simulink model "FA_18_Model"  (R2018a)
settings: Solver=ode45  StartTime=0.0  StopTime=20  FixedStep=0.1  MaxStep=0.1  RelTol=1e-3
PreLoadFcn:
  | load('FA_18_Parameters.mat')
  | format long
undefined symbols (not defined in the file or in its folder): Earth, WGS84
libraries: aerolibfltsims x1, aerolibtransform2 x1, aerolibconvert2 x1
settings Model: Creator=User  LastModifiedBy=User

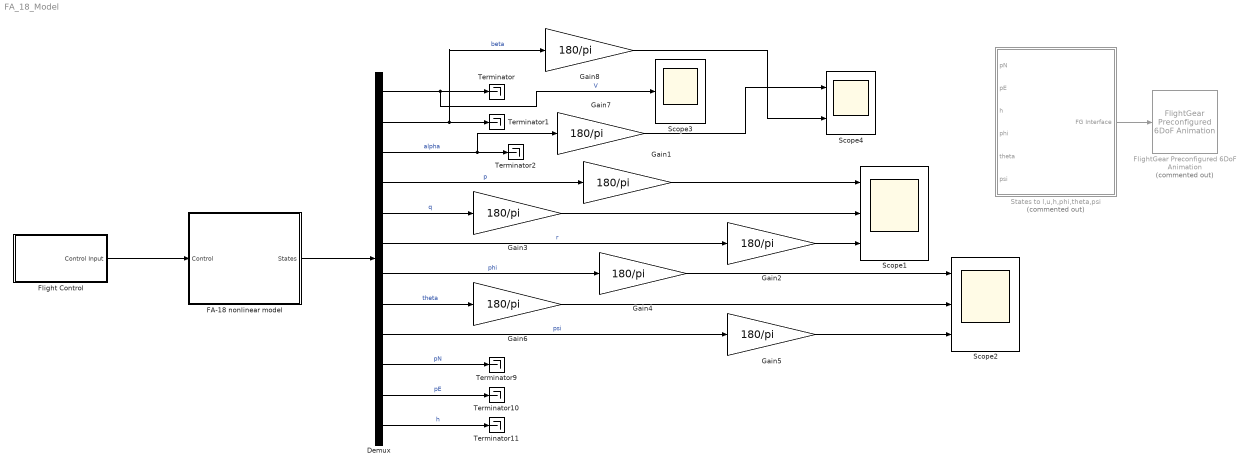
== system FA_18_Model ==
  Demux : Demux  Outputs=12
  FA-18 nonlinear model : Subsystem
  Flight Control : Subsystem
  FlightGear Preconfigured 6DoF Animation : aerolibfltsims/FlightGear Preconfigured 6DoF Animation  Commented=on  xFlightGearVersion=v2017.3  DestinationIpAddress=127.0.0.1  DestinationPort=5502  SampleTime=1/30
      settings: SourceProductName=Aerospace Blockset
  Gain{1..8} (8 alike) : Gain  Gain=180/pi
  Scope1 : Scope  NumInputPorts=3
  Scope2 : Scope  NumInputPorts=3
  Scope3 : Scope
  Scope4 : Scope  NumInputPorts=2
  States to l,u,h,phi,theta,psi : Subsystem  Commented=on
  Terminator{,1..2,9..11} (6 alike) : Terminator
  wires:
  States to l,u,h,phi,theta,psi/1(FG Interface) -> FlightGear Preconfigured 6DoF Animation/1
  Demux/3 -> Gain7/1, Terminator2/1  "alpha"
  Demux/2 -> Terminator1/1, Gain8/1  "beta"
  Demux/1 -> Scope3/1, Terminator/1  "V"
  Demux/7 -> Gain4/1  "phi"
  Demux/4 -> Gain1/1  "p"
  Demux/10 -> Terminator9/1  "pN"
  FA-18 nonlinear model/1(States) -> Demux/1
  Demux/11 -> Terminator10/1  "pE"
  Demux/6 -> Gain2/1  "r"
  Demux/12 -> Terminator11/1  "h"
  Demux/5 -> Gain3/1  "q"
  Gain1/1 -> Scope1/1
  Gain2/1 -> Scope1/3
  Gain3/1 -> Scope1/2
  Gain4/1 -> Scope2/1
  Gain5/1 -> Scope2/3
  Gain6/1 -> Scope2/2
  Demux/8 -> Gain6/1  "theta"
  Demux/9 -> Gain5/1  "psi"
  Flight Control/1(Control Input) -> FA-18 nonlinear model/1(Control)
  Gain7/1 -> Scope4/1
  Gain8/1 -> Scope4/2

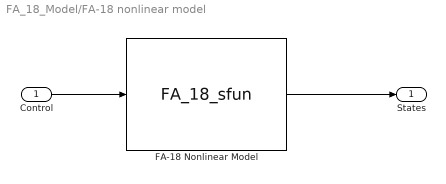
== system FA_18_Model/FA-18 nonlinear model ==
  Control : Inport
  FA-18 Nonlinear Model : S-Function  FunctionName=FA_18_sfun  SFunctionDeploymentMode=off  EnableBusSupport=off
  States : Outport
  wires:
  FA-18 Nonlinear Model/1 -> States/1
  Control/1 -> FA-18 Nonlinear Model/1

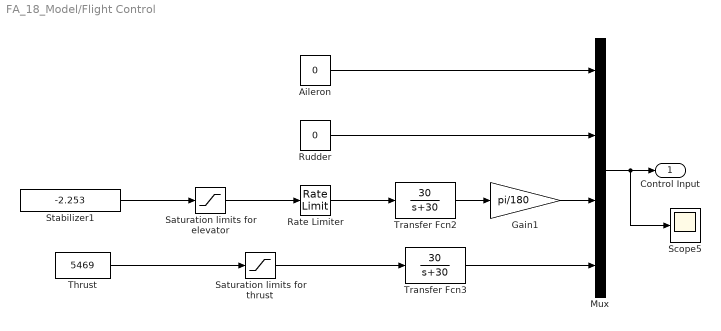
== system FA_18_Model/Flight Control ==
  Aileron : Constant  Value=0
  Gain1 : Gain  Gain=pi/180
  Mux : Mux
  Rate Limiter : RateLimiter  RisingSlewLimit=40  FallingSlewLimit=-40  SampleTimeMode=inherited
  Rudder : Constant  Value=0
  Saturation limits for elevator : Saturate  UpperLimit=10.5  LowerLimit=-24
  Saturation limits for thrust : Saturate  UpperLimit=20000  LowerLimit=0
  Scope5 : Scope
  Stabilizer1 : Constant  Value=-2.253
  Thrust : Constant  Value=5469
  Transfer Fcn2 : TransferFcn  Numerator=[30]  Denominator=[1 30]
  Transfer Fcn3 : TransferFcn  Numerator=[30]  Denominator=[1 30]
  Control Input : Outport
  wires:
  Mux/1 -> Scope5/1, Control Input/1
  Aileron/1 -> Mux/1
  Thrust/1 -> Saturation limits for thrust/1
  Transfer Fcn3/1 -> Mux/4
  Rudder/1 -> Mux/2
  Saturation limits for thrust/1 -> Transfer Fcn3/1
  Saturation limits for elevator/1 -> Rate Limiter/1
  Rate Limiter/1 -> Transfer Fcn2/1
  Stabilizer1/1 -> Saturation limits for elevator/1
  Gain1/1 -> Mux/3
  Transfer Fcn2/1 -> Gain1/1

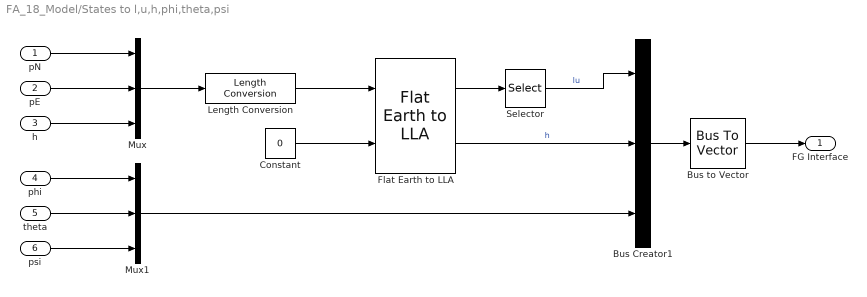
== system FA_18_Model/States to l,u,h,phi,theta,psi ==
  pN : Inport
  pE : Inport  Port=2
  h : Inport  Port=3
  phi : Inport  Port=4
  theta : Inport  Port=5
  psi : Inport  Port=6
  Bus Creator1 : BusCreator  Inputs=3
  Bus to Vector : BusToVector
  Constant : Constant  Value=0
  Flat Earth to LLA : aerolibtransform2/Flat Earth to LLA  units=Metric (MKS)  ptype=Earth (WGS84)  F=1/298.257223563  R=6378137  LL0=[50.1018 14.2632]  psi=0
  Length Conversion : aerolibconvert2/Length Conversion  IU=ft  OU=m
  Mux : Mux  Inputs=3
  Mux1 : Mux  Inputs=3
  Selector : Selector  IndexMode=Zero-based  InputPortWidth=2  IndexOptions=Index vector (dialog)  Indices=[1 0]  OutputSizes=1
  FG Interface : Outport
  wires:
  Constant/1 -> Flat Earth to LLA/2
  Length Conversion/1 -> Flat Earth to LLA/1
  Bus to Vector/1 -> FG Interface/1
  Bus Creator1/1 -> Bus to Vector/1
  Flat Earth to LLA/1 -> Selector/1
  Selector/1 -> Bus Creator1/1  "lu"
  Flat Earth to LLA/2 -> Bus Creator1/2  "h"
  pN/1 -> Mux/1
  pE/1 -> Mux/2
  h/1 -> Mux/3
  Mux/1 -> Length Conversion/1
  theta/1 -> Mux1/2
  phi/1 -> Mux1/1
  psi/1 -> Mux1/3
  Mux1/1 -> Bus Creator1/3
